simulink model "observerControl"  (Simulink 8.4)
settings: Solver=ode45  StartTime=0.0  StopTime=10.0  RelTol=1e-3
settings Model: Creator=eiseles  LastModifiedBy=eiseles
settings DataIOCC: SignalLoggingSaveFormat=Dataset
settings OptimizationCC: ExpressionDepthLimit=128
settings DebuggingCC: FcnCallInpInsideContextMsg=EnableAllAsError
settings GRTTargetCC: CombineOutputUpdateFcns=on  GRTInterface=off

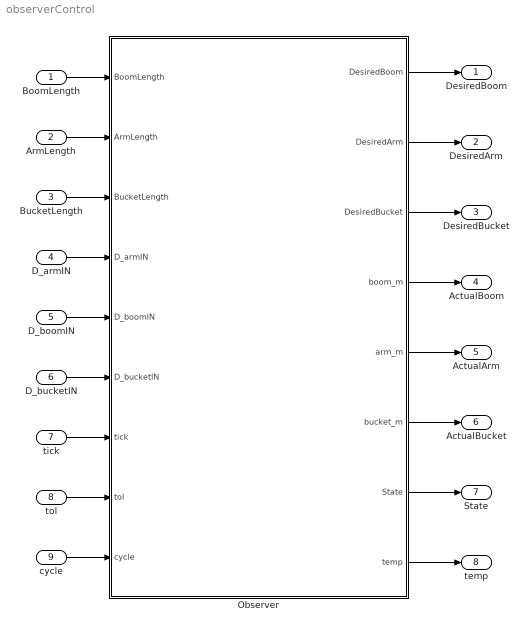
== system observerControl ==
  BoomLength : Inport
  ArmLength : Inport  Port=2
  BucketLength : Inport  Port=3
  D_armIN : Inport  Port=4
  D_boomIN : Inport  Port=5
  D_bucketIN : Inport  Port=6
  tick : Inport  Port=7
  tol : Inport  Port=8
  cycle : Inport  Port=9
  Observer : Stateflow chart  TreatAsAtomicUnit=on
  DesiredBoom : Outport
  DesiredArm : Outport  Port=2
  DesiredBucket : Outport  Port=3
  ActualBoom : Outport  Port=4
  ActualArm : Outport  Port=5
  ActualBucket : Outport  Port=6
  State : Outport  Port=7
  temp : Outport  Port=8
  wires:
  ArmLength/1 -> Observer/2(ArmLength)
  BoomLength/1 -> Observer/1(BoomLength)
  BucketLength/1 -> Observer/3(BucketLength)
  D_armIN/1 -> Observer/4(D_armIN)
  D_boomIN/1 -> Observer/5(D_boomIN)
  D_bucketIN/1 -> Observer/6(D_bucketIN)
  tick/1 -> Observer/7(tick)
  Observer/1(DesiredBoom) -> DesiredBoom/1
  Observer/2(DesiredArm) -> DesiredArm/1
  Observer/3(DesiredBucket) -> DesiredBucket/1
  Observer/4(boom_m) -> ActualBoom/1
  Observer/5(arm_m) -> ActualArm/1
  Observer/6(bucket_m) -> ActualBucket/1
  Observer/7(State) -> State/1
  Observer/8(temp) -> temp/1
  tol/1 -> Observer/8(tol)
  cycle/1 -> Observer/9(cycle)

== stateflow chart Observer ==
  state intial
    en:
    temp = -1;
    State = 0;
    DesiredBoom = D_boomIN;
    DesiredArm = D_armIN;
    DesiredBucket = D_bucketIN;
    during:boom_m = BoomLength;
    arm_m = ArmLength;
    bucket_m = BucketLength;
    DesiredBoom = D_boomIN;
    DesiredArm = D_armIN;
    DesiredBucket = D_bucketIN;
  state ready
    en:
    temp = 1;
    boom_m = BoomLength;
    arm_m = ArmLength;
    bucket_m = BucketLength;
    during:boom_m = BoomLength;
    arm_m = ArmLength;
    bucket_m = BucketLength;
  state transition
    entry:
    temp = 0;
    boom_m = BoomLength;
    arm_m = ArmLength;
    bucket_m = BucketLength;
    DesiredBoom = D_boomIN;
    DesiredArm = D_armIN;
    DesiredBucket = D_bucketIN;
    during:boom_m = BoomLength;
    arm_m = ArmLength;
    bucket_m = BucketLength;
    DesiredBoom = D_boomIN;
    DesiredArm = D_armIN;
    DesiredBucket = D_bucketIN;
  transition -> ready : [arm_m >= DesiredArm - tol  &&...
      |  arm_m <= DesiredArm +tol  &&...
      |  boom_m >= DesiredBoom -tol &&...
      |  boom_m <= DesiredBoom +tol &&...
      |  bucket_m >= DesiredBucket -tol && ...
      |  bucket_m <= DesiredBucket + tol]
      | /State = State + 1;
  ready -> ready [order 2] : [cycle==1]/State = 1;
  ready -> transition [order 1] : [(DesiredBoom != D_boomIN ||...
      |   DesiredArm != D_armIN ||...
      |   DesiredBucket != D_bucketIN)]
  intial -> transition : [arm_m >= DesiredArm - tol  &&...
      |  arm_m <= DesiredArm +tol  &&...
      |  boom_m >= DesiredBoom -tol &&...
      |  boom_m <= DesiredBoom +tol &&...
      |  bucket_m >= DesiredBucket -tol && ...
      |  bucket_m <= DesiredBucket + tol]
  (default) -> intial
  data: BoomLength input double; ArmLength input double; BucketLength input double; D_armIN input double; D_boomIN input double; D_bucketIN input double; tick input double; DesiredBoom output double; DesiredArm output double; DesiredBucket output double; boom_m output double; arm_m output double; bucket_m output double; State output double; temp output double; tol input double; cycle input double
